simulink model "directFormII_e1"  (R2014b)
settings: Solver=ode45  StartTime=0.0  StopTime=10.0  RelTol=1e-3
settings Model: Creator=ravoson  LastModifiedBy=ravoson

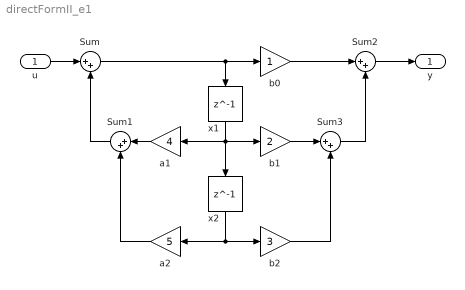
== system directFormII_e1 ==
  u : Inport
  Sum{,1..3} (4 alike) : Sum  Inputs=|++
  a1 : Gain  Gain=4
  a2 : Gain  Gain=5
  b0 : Gain
  b1 : Gain  Gain=2
  b2 : Gain  Gain=3
  x1 : Delay  DelayLength=1  InitialCondition=0
  x2 : Delay  DelayLength=1  InitialCondition=0
  y : Outport
  wires:
  u/1 -> Sum/1
  Sum/1 -> x1/1, b0/1
  Sum1/1 -> Sum/2
  b0/1 -> Sum2/1
  Sum2/1 -> y/1
  Sum3/1 -> Sum2/2
  a1/1 -> Sum1/1
  x1/1 -> x2/1, a1/1, b1/1
  b1/1 -> Sum3/1
  x2/1 -> a2/1, b2/1
  a2/1 -> Sum1/2
  b2/1 -> Sum3/2
